simulink model "simul"  (R2023a)
settings: Solver=VariableStepAuto  StartTime=0.0  StopTime=10.0  RelTol=1e-3
libraries: simulink x2
settings Model: Creator=a2408732  LastModifiedBy=a2408732

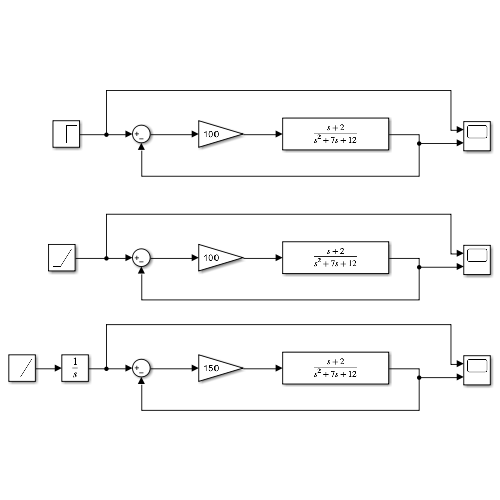
[thumbnail: Simulink's stored preview of the top-level diagram]
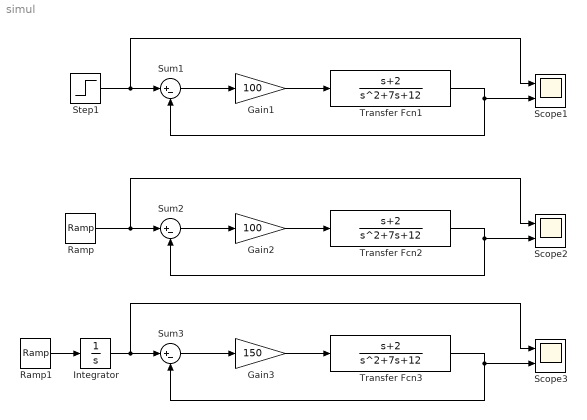
== system simul ==
  Gain1 : Gain  Gain=100
  Gain2 : Gain  Gain=100
  Gain3 : Gain  Gain=150
  Integrator : Integrator
  Ramp : simulink/Sources/Ramp  slope=1  start=0  InitialOutput=0
  Ramp1 : simulink/Sources/Ramp  slope=1  start=0  InitialOutput=0
  Scope1 : Scope  NumInputPorts=2
  Scope2 : Scope  NumInputPorts=2
  Scope3 : Scope  NumInputPorts=2
  Step1 : Step  SampleTime=0
  Sum1 : Sum  Inputs=|+-
  Sum2 : Sum  Inputs=|+-
  Sum3 : Sum  Inputs=|+-
  Transfer Fcn1 : TransferFcn  Numerator=[1 2]  Denominator=[1 7 12]
  Transfer Fcn2 : TransferFcn  Numerator=[1 2]  Denominator=[1 7 12]
  Transfer Fcn3 : TransferFcn  Numerator=[1 2]  Denominator=[1 7 12]
  wires:
  Transfer Fcn1/1 -> Sum1/2, Scope1/2
  Gain1/1 -> Transfer Fcn1/1
  Sum1/1 -> Gain1/1
  Step1/1 -> Scope1/1, Sum1/1
  Sum2/1 -> Gain2/1
  Gain2/1 -> Transfer Fcn2/1
  Transfer Fcn2/1 -> Sum2/2, Scope2/2
  Ramp/1 -> Scope2/1, Sum2/1
  Ramp1/1 -> Integrator/1
  Transfer Fcn3/1 -> Sum3/2, Scope3/2
  Sum3/1 -> Gain3/1
  Gain3/1 -> Transfer Fcn3/1
  Integrator/1 -> Scope3/1, Sum3/1
